simulink model "Model"  (R2015a)
settings: Solver=ode45  StartTime=0.0  StopTime=10.0  RelTol=1e-3
values from neighbouring files (symbols this model uses):
  Il = 0.005    [Course_Project.m]    (also in DCM.m = 0.004)
  Kb = 0.1    [Course_Project.m]    (also in DCM.m = 0.28)
  Kt = 0.1    [Course_Project.m]    (also in DCM.m = 0.25)
  L = 0.2    [Course_Project.m]    (also in DCM.m = 0.3)
  R = 1    [Course_Project.m]    (also in DCM.m = 1.1)
settings Model: Creator=user  LastModifiedBy=user

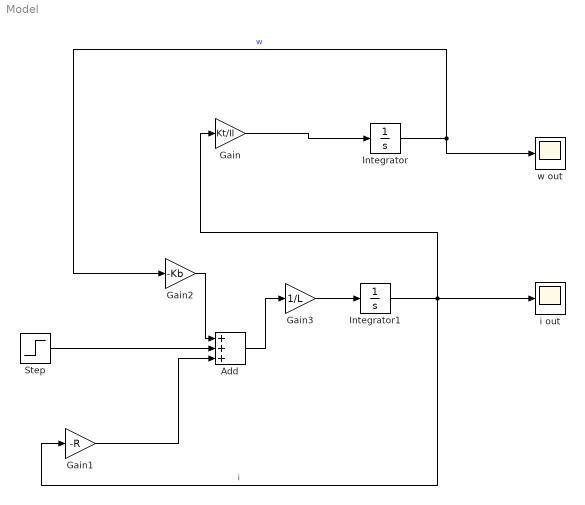
== system Model ==
  Add : Sum  Inputs=+++
  Gain : Gain  Gain=Kt/Il
  Gain1 : Gain  Gain=-R
  Gain2 : Gain  Gain=-Kb
  Gain3 : Gain  Gain=1/L
  Integrator : Integrator
  Integrator1 : Integrator
  Step : Step  SampleTime=0
  i out : Scope
  w out : Scope
  wires:
  Integrator/1 -> w out/1, Gain2/1  "w"
  Integrator1/1 -> Gain1/1, i out/1, Gain/1  "i"
  Gain/1 -> Integrator/1
  Gain2/1 -> Add/1
  Gain1/1 -> Add/3
  Add/1 -> Gain3/1
  Gain3/1 -> Integrator1/1
  Step/1 -> Add/2
